simulink model "cruise_control_002_pid"  (R2019b)
settings: Solver=VariableStepAuto  StartTime=0.0  StopTime=10.0  RelTol=1e-3
undefined symbols (not defined in the file): b, Ki, Kp, m
settings Model: Creator=Yinglongli  LastModifiedBy=Yinglongli

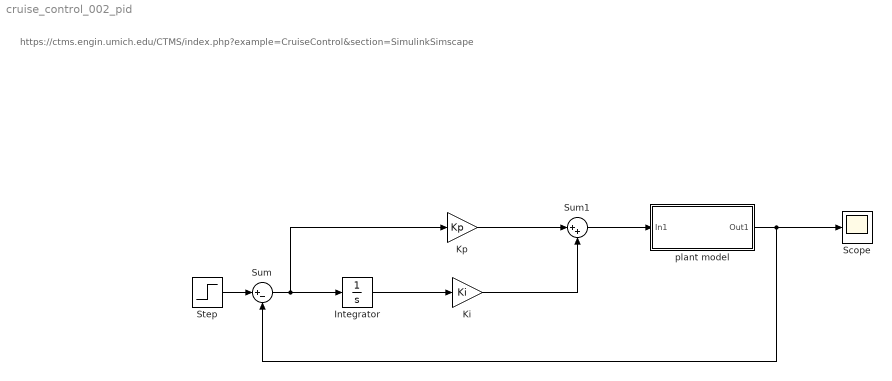
== system cruise_control_002_pid ==
  note: https://ctms.engin.umich.edu/CTMS/index.php?example=CruiseControl&section=SimulinkSimscape
  Integrator : Integrator
  Ki : Gain  Gain=Ki
  Kp : Gain  Gain=Kp
  Scope : Scope
  Step : Step  Time=0  After=u  SampleTime=0
  Sum : Sum  Inputs=|+-
  Sum1 : Sum  Inputs=|++
  "plant model " : Subsystem
  wires:
  "plant model "/1(Out1) -> Sum/2, Scope/1
  Integrator/1 -> Ki/1
  Sum/1 -> Kp/1, Integrator/1
  Kp/1 -> Sum1/1
  Ki/1 -> Sum1/2
  Sum1/1 -> "plant model "/1(In1)
  Step/1 -> Sum/1

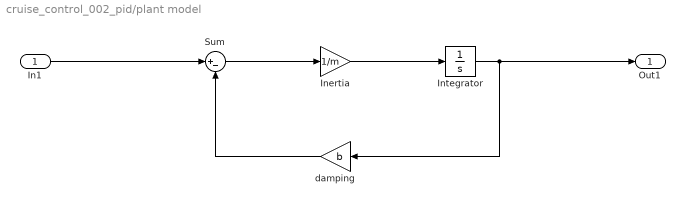
== system cruise_control_002_pid/plant model  ==
  In1 : Inport
  Inertia : Gain  Gain=1/m
  Integrator : Integrator
  Sum : Sum  Inputs=|+-
  damping : Gain  Gain=b
  Out1 : Outport
  wires:
  Inertia/1 -> Integrator/1
  Integrator/1 -> Out1/1, damping/1
  In1/1 -> Sum/1
  damping/1 -> Sum/2
  Sum/1 -> Inertia/1
